simulink model "RC_sim"  (R2022b)
settings: Solver=VariableStepAuto  StartTime=0.0  StopTime=100  FixedStep=1e-3  RelTol=1e-3
values from neighbouring files (symbols this model uses):
  C = 100 * 10^(-6)    (= 0.0001)    [RC_script.m]
  R = 5    [RC_script.m]
settings Model: Creator=brbar  LastModifiedBy=brbar

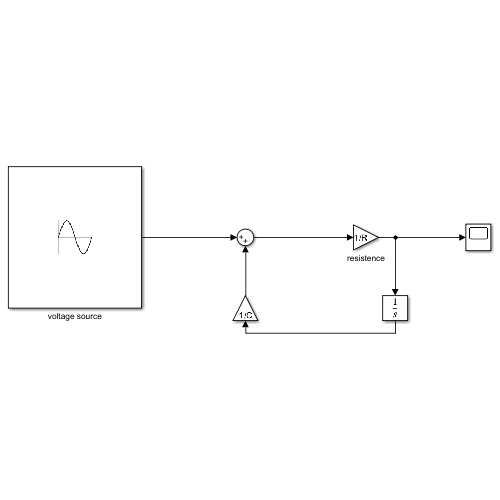
[thumbnail: Simulink's stored preview of the top-level diagram]
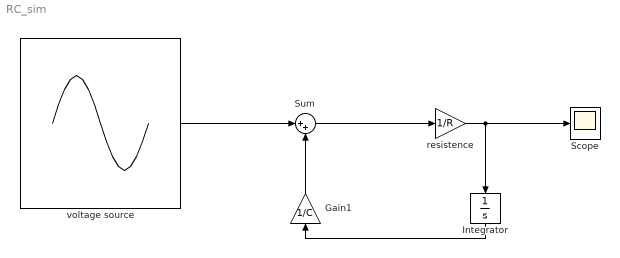
== system RC_sim ==
  Gain1 : Gain  Gain=1/C
  Integrator : Integrator
  Scope : Scope
  Sum : Sum  Inputs=|++
  resistence : Gain  Gain=1/R
  voltage source : Sin  SampleTime=0
  wires:
  voltage source/1 -> Sum/1
  Sum/1 -> resistence/1
  resistence/1 -> Integrator/1, Scope/1
  Integrator/1 -> Gain1/1
  Gain1/1 -> Sum/2
